simulink model "Exo_Origianl"  (R2023b)
settings: Solver=ode5  StartTime=0.0  StopTime=inf  FixedStep=dt  RelTol=1e-3  EnableMultiTasking=on
values from neighbouring files (symbols this model uses):
  A_0_a = 4.011    [Operator.m]
  A_0_h = 40.69    [Operator.m]
  A_0_k = 25.7    [Operator.m]
  A_1_a = 5.292    [Operator.m]
  A_1_h = 23.22    [Operator.m]
  A_1_k = -3.827    [Operator.m]
  A_2_a = -8.582    [Operator.m]
  A_2_h = -4.487    [Operator.m]
  A_2_k = -8.543    [Operator.m]
  A_3_a = -0.4755    [Operator.m]
  A_3_h = 0.3995    [Operator.m]
  A_3_k = 1.913    [Operator.m]
  A_4_a = 1.688    [Operator.m]
  A_4_k = 1.087    [Operator.m]
  A_5_a = -0.03504    [Operator.m]
  A_5_k = 2.054    [Operator.m]
  A_6_a = 1.298    [Operator.m]
  A_6_k = -0.3061    [Operator.m]
  amplitude = 0.8    [Operator.m]
  ankleStrategyInterval = 1.5    [Operator.m]
  B_1_a = 3.613    [Operator.m]
  B_1_h = -8.65    [Operator.m]
  B_1_k = -19.28    [Operator.m]
  B_2_a = -5.954    [Operator.m]
  B_2_h = 3.338    [Operator.m]
  B_2_k = 17.93    [Operator.m]
  B_3_a = 5.918    [Operator.m]
  B_3_h = 1.389    [Operator.m]
  B_3_k = 3.772    [Operator.m]
  B_4_a = -2.118    [Operator.m]
  B_4_k = 1.504    [Operator.m]
  B_5_a = 1.023    [Operator.m]
  B_5_k = 0.5838    [Operator.m]
  B_6_a = -0.7245    [Operator.m]
  B_6_k = -0.8958    [Operator.m]
  DCM_filter = 1 - dt/(dt+RC)    (= 0.926612305411)    [Operator.m]
  dt = 0.01    [Operator.m]
  frequency = 1.2    [Operator.m]
  gamma = fzero(eqn, 0.1)    [Operator.m]
  hipOffset = -17    [Operator.m]
  K_high = 0.5    [Operator.m]
  K_low = 0.5    [Operator.m]
  KD = 0.39    [Operator.m]
  Kp = 10    [Operator.m]
  l3 = userHeight*0.232    (= 15.776)    [Operator.m]
  l4 = userHeight*0.247    (= 16.796)    [Operator.m]
  l_c2 = ((0.29*34.66+0.63*6.07)/(6.07+34.66))/(0.52+0.19)*l2    (= 15.0425832454)    [Operator.m]
  l_c3 = 0.17/0.40*l3    (= 6.7048)    [Operator.m]
  l_c4 = ((0.19*3.52+0.43*1.05)/(3.52+1.05))/0.43*l4    (= 9.57536959951)    [Operator.m]
  l_foot = 11.25    [Operator.m]
  m2 = m2 + 2.2048*7.591    (= 119.8566368)    [Operator.m]
  m3 = m3 + 2.2048*1.715    (= 19.781232)    [Operator.m]
  m4 = userWeight*(0.0459+0.0169)    (= 10.048)    [Operator.m]
  m_Exo = 2.2048*1.647    (= 3.6313056)    [Operator.m]
  m_f = userWeight*0.0169    (= 2.704)    [Operator.m]
  maxTorque = 35    [Operator.m]
  P_t_ZMP_gain_Ankle = 0    [Operator.m]
  P_t_ZMP_gain_Hip = 0    [Operator.m]
  Phase_Left = 2+pi    (= 5.14159265359)    [Operator.m]
  Phase_Right = 2    [Operator.m]
  ramp = 2    [Operator.m]
  Strategy_filter = DCM_filter    (= 0.926612305411)    [Operator.m]
  strategySaturation = 10    [Operator.m]
  userHeight = 68    [Operator.m]
  userWeight = 160    [Operator.m]
undefined symbols (not defined in the file or in its folder): CAN_Device, DCMErrorPenalty, PEAK, Phase_Left_Knee_0, System, totalPowerPenalty
libraries: sldrtlib x35, simulink x16, rllib x1
(part 4 of 4)

== matlab function Exo_Origianl/If Action Subsystem3/Subsystem7/MATLAB Function ==
  data: u input; y output
function y = fcn(u)
    if isempty(u) || isnan(u)
        y = 0;
    else
        y = u;
    end
end

== matlab function Exo_Origianl/If Action Subsystem3/Subsystem/MATLAB Function ==
  data: u input; y output
function y = fcn(u)
    if isempty(u) || isnan(u)
        y = 0;
    else
        y = u;
    end
end

== matlab function Exo_Origianl/If Action Subsystem3/Subsystem/MATLAB Function2 ==
  data: u input; y output
function y = fcn(u)
    if isempty(u) || isnan(u)
        y = 0;
    else
        y = u;
    end
end

== matlab function Exo_Origianl/If Action Subsystem3/Subsystem/MATLAB Function5 ==
  data: alpha input; u input; y_delay input; y output
function y = fcn(alpha, u, y_delay)
y = alpha*y_delay + (1-alpha)*u;

== matlab function Exo_Origianl/If Action Subsystem3/Subsystem7/Initialization ==
  settings: updateMethod=DISCRETE
  data: clock input; TimeUp output; trigger input; ramp input; TimeDown output
function [TimeUp, TimeDown] = resetTimer(clock, trigger, ramp)
    persistent lastTriggerTime prevTrigger;
    if isempty(lastTriggerTime)
        lastTriggerTime = 0;
    end
    if isempty(prevTrigger)
        prevTrigger = 0;
    end

    if trigger == 1 && prevTrigger ~= 1
        lastTriggerTime = clock;
    end

    prevTrigger = trigger;

    TimeDown = 1 - 1/ramp*(clock - lastTriggerTime);
    TimeUp = 1/ramp*(clock - lastTriggerTime);
end

== matlab function Exo_Origianl/If Action Subsystem3/Subsystem7/MATLAB Function1 ==
  data: u input; y output
function y = fcn(u)
    if isempty(u) || isnan(u)
        y = 0;
    else
        y = u;
    end
end

== matlab function Exo_Origianl/If Action Subsystem3/Subsystem7/MATLAB Function3 ==
  data: u input; y output
function y = fcn(u)
    if isempty(u) || isnan(u)
        y = 0;
    else
        y = u;
    end
end

== matlab function Exo_Origianl/If Action Subsystem3/Subsystem7/MATLAB Function5 ==
  data: alpha input; u input; y_delay input; y output
function y = fcn(alpha, u, y_delay)
y = alpha*y_delay + (1-alpha)*u;

== matlab function Exo_Origianl/If Action Subsystem3/Subsystem2/Step Tracking ==
  settings: updateMethod=DISCRETE
  data: currentStep output; stepTime output; rightStep input; leftStep input; currentTime input; frequency input; ankleStrategyInterval input
function [currentStep, stepTime] = stepTracking(rightStep, leftStep, currentTime, frequency, ankleStrategyInterval)
    frequency = frequency*2;
    T = 2*pi/frequency;
    stepDuration = ankleStrategyInterval*T;

    % Define persistent variables
    persistent lastInput;
    persistent lastUpdateTime;
    persistent previousStep;
    
    % Initialize default values
    if isempty(lastInput)
        lastInput = 0;
    end
    if isempty(lastUpdateTime)
        lastUpdateTime = 0;
    end
    if isempty(previousStep)
        previousStep = 0;
    end

    % Check which input was triggered most recently
    if rightStep == 1 && leftStep == 0
        lastInput = 1; % Indicates that rightStep was triggered last
    elseif leftStep == 1 && rightStep == 0
        lastInput = -1; % Indicates that leftStep was triggered last
    end

    % Update the current step
    currentStep = lastInput;
    
    % Reset lastUpdateTime if currentStep changes
    if currentStep ~= previousStep
        lastUpdateTime = currentTime;
    end

    % Calculate time since the last trigger
    stepTime = currentTime - lastUpdateTime;

    % Reset currentStep to 0 if stepDuration has passed
    if stepTime >= stepDuration
        currentStep = 0;
    end

    % Update previous step
    previousStep = currentStep;
end

== matlab function Exo_Origianl/If Action Subsystem3/Subsystem7/MATLAB Function4 ==
  data: alpha input; u input; y_delay input; y output
function y = fcn(alpha, u, y_delay)
y = alpha*y_delay + (1-alpha)*u;

== matlab function Exo_Origianl/If Action Subsystem3/Subsystem7/MATLAB Function6 ==
  data: alpha input; u input; y_delay input; y output
function y = fcn(alpha, u, y_delay)
y = alpha*y_delay + (1-alpha)*u;

== matlab function Exo_Origianl/If Action Subsystem3/Subsystem1/MATLAB Function ==
  data: u input; y output
function y = fcn(u)
    if isempty(u) || isnan(u)
        y = 0;
    else
        y = u;
    end
end

== matlab function Exo_Origianl/If Action Subsystem3/Subsystem7/MATLAB Function2 ==
  data: u input; K_high output; K_low output
function [K_high, K_low] = fcn(u)
    if u == 1
        K_high = 0;
        K_low = 1;
    else
        K_high = 1;
        K_low = 0;
end

== matlab function Exo_Origianl/If Action Subsystem3/Pressure filtering/MATLAB Function5 ==
  data: alpha input; u input; y_delay input; y output
function y = fcn(alpha, u, y_delay)
y = alpha*y_delay + (1-alpha)*u;

== matlab function Exo_Origianl/If Action Subsystem3/Pressure filtering/MATLAB Function1 ==
  data: alpha input; u input; y_delay input; y output
function y = fcn(alpha, u, y_delay)
y = alpha*y_delay + (1-alpha)*u;

== matlab function Exo_Origianl/If Action Subsystem3/Pressure filtering/MATLAB Function2 ==
  data: alpha input; u input; y_delay input; y output
function y = fcn(alpha, u, y_delay)
y = alpha*y_delay + (1-alpha)*u;

== matlab function Exo_Origianl/If Action Subsystem3/Pressure filtering/MATLAB Function3 ==
  data: alpha input; u input; y_delay input; y output
function y = fcn(alpha, u, y_delay)
y = alpha*y_delay + (1-alpha)*u;

== matlab function Exo_Origianl/If Action Subsystem3/Subsystem7/MATLAB Function7 ==
  data: alpha input; u input; y_delay input; y output
function y = fcn(alpha, u, y_delay)
y = alpha*y_delay + (1-alpha)*u;

== matlab function Exo_Origianl/If Action Subsystem3/Subsystem7/MATLAB Function8 ==
  data: alpha input; u input; y_delay input; y output
function y = fcn(alpha, u, y_delay)
y = alpha*y_delay + (1-alpha)*u;

== matlab function Exo_Origianl/If Action Subsystem3/Subsystem7/MATLAB Function9 ==
  data: alpha input; u input; y_delay input; y output
function y = fcn(alpha, u, y_delay)
y = alpha*y_delay + (1-alpha)*u;

== matlab function Exo_Origianl/If Action Subsystem3/Subsystem2/Noise filtering/MATLAB Function2 ==
  data: alpha input; u input; y_delay input; y output
function y = fcn(alpha, u, y_delay)
y = alpha*y_delay + (1-alpha)*u;

== matlab function Exo_Origianl/If Action Subsystem3/Subsystem2/Noise filtering/MATLAB Function3 ==
  data: alpha input; u input; y_delay input; y output
function y = fcn(alpha, u, y_delay)
y = alpha*y_delay + (1-alpha)*u;

== matlab function Exo_Origianl/If Action Subsystem3/Subsystem2/DCM Strategy ==
  data: RHP input; RTP input; LHP input; LTP input; Right_Hip_Desired input; Right_Knee_Desired input; Right_Ankle_Desired input; Left_Hip_Desired input; Left_Knee_Desired input; Left_Ankle_Desired input; Right_Hip_Angle input; Right_Knee_Angle input; Right_Ankle_Angle input; Left_Hip_Angle input; Left_Knee_Angle input; Left_Ankle_Angle input; x_CoM_right output; x_CoM_right_act output; alpha_right output; alpha_right_act output; x_CoM_left output; x_CoM_left_act output; alpha_left output; alpha_left_act output; CoM_Right output; m2 input; m3 input; m4 input; l_c2 input; l_c3 input; l_c4 input; m_f input; l_foot input; m_Exo input; l3 input; l4 input; CoM_Left output
function [x_CoM_right, x_CoM_right_act, alpha_right, alpha_right_act, x_CoM_left, x_CoM_left_act, alpha_left, alpha_left_act, CoM_Right, CoM_Left] = ankleStrategy(...
    RHP, RTP, LHP, LTP, ...
    Right_Hip_Desired, Right_Knee_Desired, Right_Ankle_Desired, Left_Hip_Desired, Left_Knee_Desired, Left_Ankle_Desired, ...
    Right_Hip_Angle, Right_Knee_Angle, Right_Ankle_Angle, Left_Hip_Angle, Left_Knee_Angle, Left_Ankle_Angle, ...
    m2, m3, m4, l_c2, l_c3, l_c4, m_f, l_foot, m_Exo, l3, l4)

    g = 32.1741*12; % Gravity [in/s^2]
    footLength = 8; % [in] (estimated pressure sensor location)
    M = [m_f m4 m3 m2 m3 m4 m_f m_Exo];

    % [in]
    phi = [l_foot/2 0       0       0    0    0    0        0;
           0        l4-l_c4 0       0    0    0    0        0;
           0        l4      l3-l_c3 0    0    0    0        0;
           0        l4      l3      l_c2 0    0    0        0;
           0        l4      l3      0    l_c3 0    0        0;
           0        l4      l3      0    l3   l_c4 0        0;
           0        l4      l3      0    l3   l4   l_foot/2 0;
           0        l4      l3      0    0    0    0        4.51]; % for exo battery

    % Left step (right foot on ground)
    p_right = [1;
         cosd(90-Right_Ankle_Desired);
         cosd(90-Right_Ankle_Desired + Right_Knee_Desired);
         cosd(90-Right_Ankle_Desired + Right_Knee_Desired - Right_Hip_Desired);
         -cosd(90-Right_Ankle_Desired + Right_Knee_Desired + Left_Hip_Desired - Right_Hip_Desired);
         -cosd(90-Right_Ankle_Desired + Right_Knee_Desired + Left_Hip_Desired - Right_Hip_Desired - Left_Knee_Desired);
         cosd(90-Right_Ankle_Desired + Right_Knee_Desired + Left_Hip_Desired - Right_Hip_Desired - Left_Knee_Desired - 90+Left_Ankle_Desired);
         cosd(90-Right_Ankle_Desired + Right_Knee_Desired - Right_Hip_Desired + 8.278)];

    q_right = [1;
         sind(90-Right_Ankle_Desired);
         sind(90-Right_Ankle_Desired + Right_Knee_Desired);
         sind(90-Right_Ankle_Desired + Right_Knee_Desired - Right_Hip_Desired);
         -sind(90-Right_Ankle_Desired + Right_Knee_Desired + Left_Hip_Desired - Right_Hip_Desired);
         -sind(90-Right_Ankle_Desired + Right_Knee_Desired + Left_Hip_Desired - Right_Hip_Desired - Left_Knee_Desired);
         sind(90-Right_Ankle_Desired + Right_Knee_Desired + Left_Hip_Desired - Right_Hip_Desired - Left_Knee_Desired - 90+Left_Ankle_Desired);
         sind(90-Right_Ankle_Desired + Right_Knee_Desired - Right_Hip_Desired + 8.278)];
    
    p_act_right = [1;
         cosd(90-Right_Ankle_Angle);
         cosd(90-Right_Ankle_Angle + Right_Knee_Angle);
         cosd(90-Right_Ankle_Angle + Right_Knee_Angle - Right_Hip_Angle);
         -cosd(90-Right_Ankle_Angle + Right_Knee_Angle + Left_Hip_Angle - Right_Hip_Angle);
         -cosd(90-Right_Ankle_Angle + Right_Knee_Angle + Left_Hip_Angle - Right_Hip_Angle - Left_Knee_Angle);
         cosd(90-Right_Ankle_Angle + Right_Knee_Angle + Left_Hip_Angle - Right_Hip_Angle - Left_Knee_Angle - 90+Left_Ankle_Angle);
         cosd(90-Right_Ankle_Angle + Right_Knee_Angle - Right_Hip_Angle + 8.278)];

    q_act_right = [1;
         sind(90-Right_Ankle_Angle);
         sind(90-Right_Ankle_Angle + Right_Knee_Angle);
         sind(90-Right_Ankle_Angle + Right_Knee_Angle - Right_Hip_Angle);
         -sind(90-Right_Ankle_Angle + Right_Knee_Angle + Left_Hip_Angle - Right_Hip_Angle);
         -sind(90-Right_Ankle_Angle + Right_Knee_Angle + Left_Hip_Angle - Right_Hip_Angle - Left_Knee_Angle);
         sind(90-Right_Ankle_Angle + Right_Knee_Angle + Left_Hip_Angle - Right_Hip_Angle - Left_Knee_Angle - 90+Left_Ankle_Angle);
         sind(90-Right_Ankle_Angle + Right_Knee_Angle - Right_Hip_Angle + 8.278)];

    x_CoM_right = M*phi*p_right/sum(M); % - (footLength*RTP + phi(7,:)*p_right*LHP + (phi(7,:)*p_right+footLength/2)*LTP)/(RHP + RTP + LHP + LTP);
    x_CoM_right_act = M*phi*p_act_right/sum(M); % - (footLength*RTP + phi(7,:)*p_act_right*LHP + (phi(7,:)*p_act_right+footLength/2)*LTP)/(RHP + RTP + LHP + LTP);

    alpha_right = g/(M*phi*q_right/sum(M));
    alpha_right_act = g/(M*phi*q_act_right/sum(M));

    CoM_Right = (footLength*RTP + phi(7,:)*p_right*LHP + (phi(7,:)*p_right+footLength/2)*LTP)/(RHP + RTP + LHP + LTP);


    % Right step (left foot on ground)
    p_left = [1;
         cosd(90-Left_Ankle_Desired);
         cosd(90-Left_Ankle_Desired + Left_Knee_Desired);
         cosd(90-Left_Ankle_Desired + Left_Knee_Desired - Left_Hip_Desired);
         -cosd(90-Left_Ankle_Desired + Left_Knee_Desired + Right_Hip_Desired - Left_Hip_Desired);
         -cosd(90-Left_Ankle_Desired + Left_Knee_Desired + Right_Hip_Desired - Left_Hip_Desired - Right_Knee_Desired);
         cosd(90-Left_Ankle_Desired + Left_Knee_Desired + Right_Hip_Desired - Left_Hip_Desired - Right_Knee_Desired - 90+Right_Ankle_Desired);
         cosd(90-Left_Ankle_Desired + Left_Knee_Desired - Left_Hip_Desired + 8.278)];

    q_left = [1;
         sind(90-Left_Ankle_Desired);
         sind(90-Left_Ankle_Desired + Left_Knee_Desired);
         sind(90-Left_Ankle_Desired + Left_Knee_Desired - Left_Hip_Desired);
         -sind(90-Left_Ankle_Desired + Left_Knee_Desired + Right_Hip_Desired - Left_Hip_Desired);
         -sind(90-Left_Ankle_Desired + Left_Knee_Desired + Right_Hip_Desired - Left_Hip_Desired - Right_Knee_Desired);
         sind(90-Left_Ankle_Desired + Left_Knee_Desired + Right_Hip_Desired - Left_Hip_Desired - Right_Knee_Desired - 90+Right_Ankle_Desired);
         sind(90-Left_Ankle_Desired + Left_Knee_Desired - Left_Hip_Desired + 8.278)];
    
    p_act_left = [1;
         cosd(90-Left_Ankle_Angle);
         cosd(90-Left_Ankle_Angle + Left_Knee_Angle);
         cosd(90-Left_Ankle_Angle + Left_Knee_Angle - Left_Hip_Angle);
         -cosd(90-Left_Ankle_Angle + Left_Knee_Angle + Right_Hip_Angle - Left_Hip_Angle);
         -cosd(90-Left_Ankle_Angle + Left_Knee_Angle + Right_Hip_Angle - Left_Hip_Angle - Right_Knee_Angle);
         cosd(90-Left_Ankle_Angle + Left_Knee_Angle + Right_Hip_Angle - Left_Hip_Angle - Right_Knee_Angle - 90+Right_Ankle_Angle);
         cosd(90-Left_Ankle_Angle + Left_Knee_Angle - Left_Hip_Angle + 8.278)];

    q_act_left = [1;
         sind(90-Left_Ankle_Angle);
         sind(90-Left_Ankle_Angle + Left_Knee_Angle);
         sind(90-Left_Ankle_Angle + Left_Knee_Angle - Left_Hip_Angle);
         -sind(90-Left_Ankle_Angle + Left_Knee_Angle + Right_Hip_Angle - Left_Hip_Angle);
         -sind(90-Left_Ankle_Angle + Left_Knee_Angle + Right_Hip_Angle - Left_Hip_Angle - Right_Knee_Angle);
         sind(90-Left_Ankle_Angle + Left_Knee_Angle + Right_Hip_Angle - Left_Hip_Angle - Right_Knee_Angle - 90+Right_Ankle_Angle);
         sind(90-Left_Ankle_Angle + Left_Knee_Angle - Left_Hip_Angle + 8.278)];

    x_CoM_left = M*phi*p_left/sum(M); % - (footLength*LTP + phi(7,:)*p_right*RHP + (phi(7,:)*p_right+footLength/2)*RTP)/(RHP + RTP + LHP + LTP);
    x_CoM_left_act = M*phi*p_act_left/sum(M); % - (footLength*LTP + phi(7,:)*p_act_right*RHP + (phi(7,:)*p_act_right+footLength/2)*RTP)/(RHP + RTP + LHP + LTP);

    alpha_left = g/(M*phi*q_left/sum(M));
    alpha_left_act = g/(M*phi*q_act_left/sum(M));

    CoM_Left = (footLength*LTP + phi(7,:)*p_left*RHP + (phi(7,:)*p_left+footLength/2)*RTP)/(RHP + RTP + LHP + LTP);
end

== matlab function Exo_Origianl/If Action Subsystem3/Subsystem2/Right Ankle Strategy ==
  data: currentStep input; frequency input; t input; gamma input; x_CoM_right input; x_CoMdot_right input; x_CoM_right_act input; x_CoMdot_right_act input; alpha_right input; P_t_ZMP_right output; alpha_right_act input; zeta_t_err output; zeta_t output; zeta_act output
function [P_t_ZMP_right, zeta_t_err, zeta_t, zeta_act] = P_t_ZMP_right(currentStep, frequency, t, gamma, x_CoM_right, x_CoMdot_right, x_CoM_right_act, x_CoMdot_right_act, alpha_right, alpha_right_act)

    frequency = frequency*2;
    T = 2*pi/frequency;

    if currentStep == 1 % left step (right foot on ground)
        if alpha_right > 0
            zeta_t = x_CoM_right + x_CoMdot_right/sqrt(alpha_right);
        else
            zeta_t = 0;
        end
        if alpha_right_act > 0
            zeta_act = x_CoM_right_act + x_CoMdot_right_act/sqrt(alpha_right_act);
        else
            zeta_act = 0;
        end
        zeta_t_err = zeta_t - zeta_act;
        %P_t_ZMP_right = exp(frequency*(T - t))/(1-exp(frequency*(T - t)) - gamma)*zeta_t_err;
        %P_t_ZMP_right = -zeta_t_err*(1+t)^(1+gamma);
        %P_t_ZMP_right = -(exp(gamma*t));
        P_t_ZMP_right = -1;

    else
        zeta_t_err = 0;
        P_t_ZMP_right = 0;
        zeta_t = 0;
        zeta_act = 0;
    end
end

== matlab function Exo_Origianl/If Action Subsystem3/Subsystem2/Left Ankle Strategy ==
  data: x_CoM_left input; x_CoMdot_left input; x_CoM_left_act input; x_CoMdot_left_act input; alpha_left input; alpha_left_act input; gamma input; currentStep input; frequency input; t input; P_t_ZMP_left output; zeta_t_err output; zeta_t output; zeta_act output
function [P_t_ZMP_left, zeta_t_err, zeta_t, zeta_act] = P_t_ZMP_left(x_CoM_left, x_CoMdot_left, x_CoM_left_act, x_CoMdot_left_act, alpha_left, alpha_left_act, gamma, currentStep, frequency, t)

    frequency = frequency*2;
    T = 2*pi/frequency;

    if currentStep == -1 % right step (left foot on ground)
        if alpha_left > 0
            zeta_t = x_CoM_left + x_CoMdot_left/sqrt(alpha_left);
        else
            zeta_t = 0;
        end
        if alpha_left_act > 0
            zeta_act = x_CoM_left_act + x_CoMdot_left_act/sqrt(alpha_left_act);
        else
            zeta_act = 0;
        end
        zeta_t_err = zeta_t - zeta_act;
        %P_t_ZMP_left = exp(frequency*(T - t))/(1-exp(frequency*(T - t)) - gamma)*zeta_t_err;
        %P_t_ZMP_left = zeta_t_err*(1+t)^(1+gamma);
        %P_t_ZMP_left = -(exp(gamma*t));
        P_t_ZMP_left = -1;

    else
        zeta_t_err = 0;
        P_t_ZMP_left = 0;
        zeta_t = 0;
        zeta_act = 0;
    end
end
